simulink library "busLib"  (Simulink 6.0)
settings: Solver=ode45  StartTime=0.0  StopTime=10.0  RelTol=1e-3
libraries: busLib x2
settings Model: Creator=awarlock  LastModifiedBy=awarlock  ExtModeAutoUpdateStatusClock=off

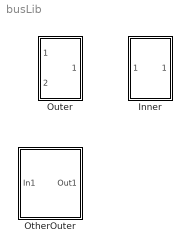
== system busLib ==
  Inner : Subsystem  TreatAsAtomicUnit=on
  OtherOuter : Subsystem  TreatAsAtomicUnit=on
  Outer : Subsystem  TreatAsAtomicUnit=on

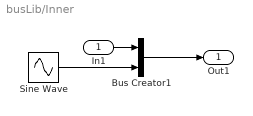
== system busLib/Inner ==
  In1 : Inport  Port=1  LatchInput=off
  Bus Creator1 : BusCreator  DialogController=Simulink.DDGSource_Bus  Inputs=2
  Sine Wave : Sin  SampleTime=0.1
  Out1 : Outport
  wires:
  In1/1 -> Bus Creator1/1
  Bus Creator1/1 -> Out1/1
  Sine Wave/1 -> Bus Creator1/2

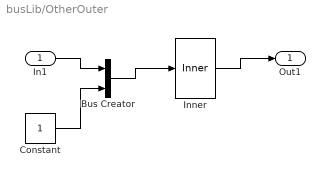
== system busLib/OtherOuter ==
  In1 : Inport  Port=1  LatchInput=off
  Bus Creator : BusCreator  DialogController=Simulink.DDGSource_Bus  Inputs=2
  Constant : Constant  SampleTime=0.1
  Inner : busLib/Inner
  Out1 : Outport
  wires:
  In1/1 -> Bus Creator/1
  Constant/1 -> Bus Creator/2
  Bus Creator/1 -> Inner/1
  Inner/1 -> Out1/1

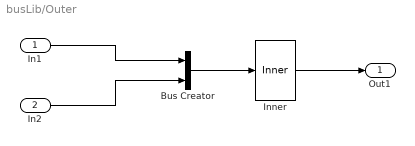
== system busLib/Outer ==
  In1 : Inport  Port=1  LatchInput=off
  In2 : Inport  Port=2  LatchInput=off
  Bus Creator : BusCreator  DialogController=Simulink.DDGSource_Bus  Inputs=2
  Inner : busLib/Inner
  Out1 : Outport
  wires:
  In1/1 -> Bus Creator/1
  In2/1 -> Bus Creator/2
  Bus Creator/1 -> Inner/1
  Inner/1 -> Out1/1
